simulink model "week1prob3"  (R2021a)
settings: Solver=VariableStepAuto  StartTime=0.0  StopTime=10.0  RelTol=1e-3
settings Model: Creator=Nida  LastModifiedBy=Nida

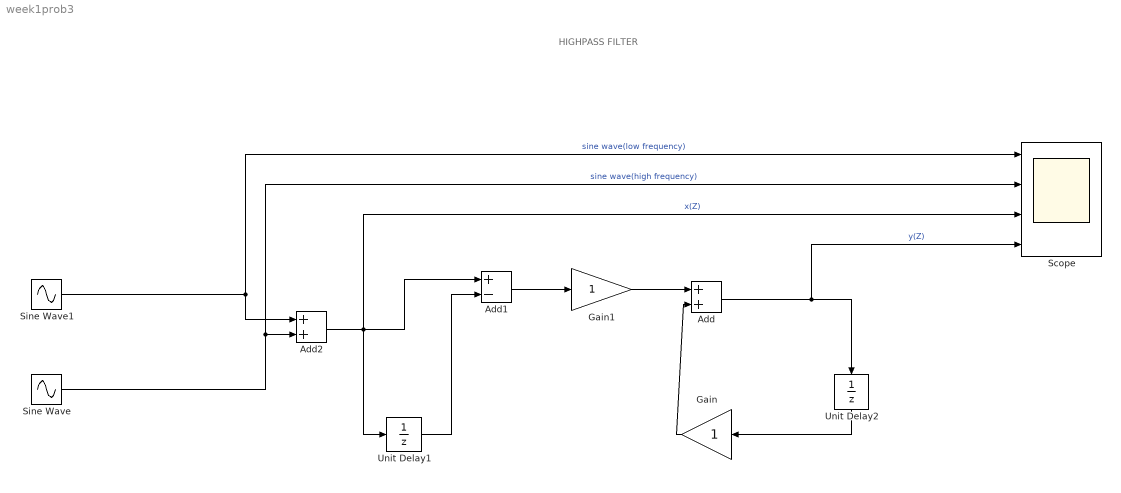
== system week1prob3 ==
  note: HIGHPASS FILTER
  Add : Sum
  Add1 : Sum  Inputs=+-
  Add2 : Sum
  Gain : Gain
  Gain1 : Gain
  Scope : Scope  NumInputPorts=4
  Sine Wave : Sin  Frequency=3000  SampleTime=0
  Sine Wave1 : Sin  Frequency=800  SampleTime=0
  Unit Delay1 : UnitDelay  SampleTime=-1  HasFrameUpgradeWarning=on
  Unit Delay2 : UnitDelay  SampleTime=-1  HasFrameUpgradeWarning=on
  wires:
  Sine Wave1/1 -> Add2/1, Scope/1  "sine wave(low frequency)"
  Add1/1 -> Gain1/1
  Gain/1 -> Add/2
  Unit Delay1/1 -> Add1/2
  Gain1/1 -> Add/1
  Add/1 -> Unit Delay2/1, Scope/4  "y(Z)"
  Sine Wave/1 -> Scope/2, Add2/2  "sine wave(high frequency)"
  Unit Delay2/1 -> Gain/1
  Add2/1 -> Scope/3, Unit Delay1/1, Add1/1  "x(Z)"
